simulink model "high_level"  (R2016b)
settings: Solver=FixedStepAuto  StartTime=0.0  StopTime=inf  FixedStep=0.05  RelTol=1e-3
values from neighbouring files (symbols this model uses):
  Ki = 0.2    [run.m]    (also in run_with_python.m)
  Kia = 20    [run.m]    (also in run_with_python.m = -0.3)
  kiax = 20    [run.m]    (also in run_with_python.m)
  Kix = 0.2    [run.m]    (also in run_with_python.m)
  Kp = 11.9    [run.m]    (also in run_with_python.m = 6)
  Kpa = 4    [run.m]    (also in run_with_python.m)
  Kpax = 4    [run.m]    (also in run_with_python.m)
  Kpx = 11.9    [run.m]    (also in run_with_python.m)
  START_COURSE = 1    [run.m]    (also in run_with_python.m)
  total_waypoints = length(xwaypoints)    [run.m]    (also in run_with_python.m = length(waypoints_list))
  TxBreak = 0    [run.m]    (also in run_with_python.m)
  TxCoulomb = 2.5    [run.m]    (also in run_with_python.m)
  TxVisc = 49.1750    (= 49.175)    [run.m]    (also in run_with_python.m)
  TyBreak = 0    [run.m]    (also in run_with_python.m)
  TyCoulomb = 1.8    [run.m]    (also in run_with_python.m)
  xwaypoints = targets(:,1)/100    [run.m]
  xZero = 0    [run.m]    (also in run_with_python.m)
  ywaypoints = targets(:,2)/100    [run.m]
  yZero = 0.    (= 0)    [run.m]    (also in run_with_python.m)
undefined symbols (not defined in the file or in its folder): m, MR, TzBreak, TzCoulomb, X, xRange, Y, yRange, Z, zRange, zZero
undefined symbols (not defined in the file): M, TorqueMultX, TorqueMultY, TorqueMultZ, TxTrans, TyTrans, TyVisc, TzTrans, TzVisc
libraries: sm_lib x146, fl_lib x62, nesl_utility x24, elec_lib x9, simulink x6, sm_double_wishbone_suspension_lib x4, aerolibtransform2 x1
(part 1 of 14)
settings Model: Creator=nadeen  LastModifiedBy=nadeen
settings DataIOCC: ReturnWorkspaceOutputs=on

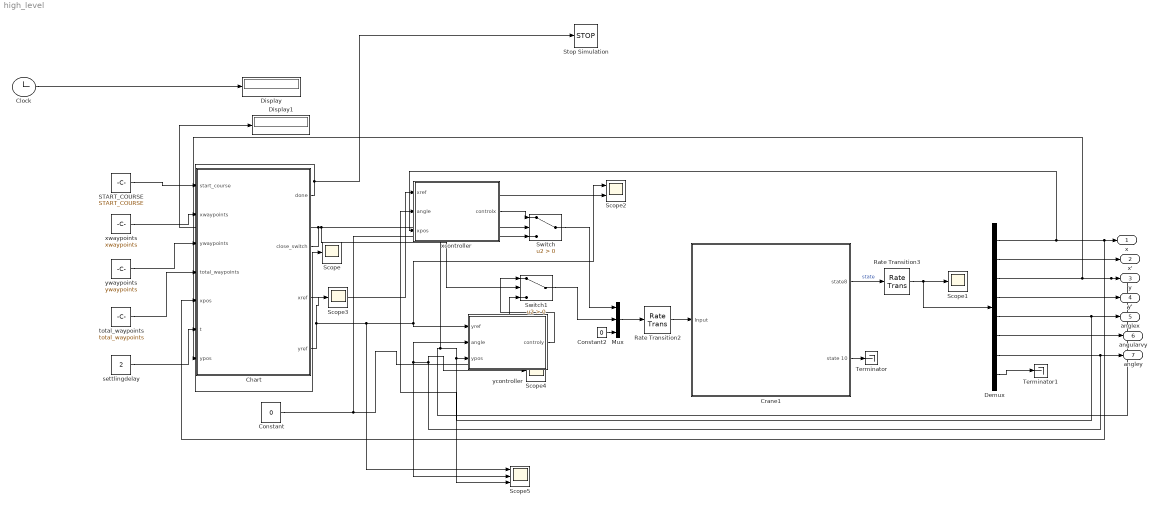
== system high_level ==
  Chart : Stateflow chart  TreatAsAtomicUnit=on
  Clock : Clock
  Constant : Constant  Value=0
  Constant2 : Constant  Value=0
  Crane1 : Subsystem  mask{penduMass=m, cartMass=M, MR=MR, xRange=xRange, yRange=yRange, zRange=zRange, xZero=xZero, yZero=yZero, zZero=zZero, TxBreak=TxBreak, TxCoulomb=TxCoulomb, TxVisc=TxVisc, TxTrans=TxTrans, TyBreak=TyBreak, TyCoulomb=TyCoulomb, TyVisc=TyVisc, TyTrans=TyTrans, TzBreak=TzBreak, TzCoulomb=TzCoulomb, TzVisc=TzVisc, TzTrans=TzTrans, Ux=TorqueMultX, Uy=TorqueMultY, Uz=TorqueMultZ}
      mask prompts: penduMass "Pendulum Mass (Kg)"; cartMass "Mass of the cart (Kg)"; MR "Mass of the rail (Kg)"; TxBreak "BreakAwayFriction"; TxCoulomb "Coulomb Friction"; TxVisc "Viscous friction"; TxTrans "Transition coeff"; TyBreak "BreakAwayFriction"; TyCoulomb "Coulomb Friction"; TyVisc "Viscous friction"; TyTrans "Transition coeff"; TzBreak "BreakAwayFriction"; TzCoulomb "Coulomb Friction"; TzVisc "Viscous friction"; TzTrans "Transition coeff"; Ux "Rail motor multiplier (X)"; Uy "Cart motor multiplier (Y)"; Uz "String motor multiplier (Z)"
      mask init:
      | %mass lowSat
      | penduMass=max(penduMass,1e-3);
      | cartMass=max(cartMass,1e-3);
      | MR=max(MR,1e-3);
      | 
      | %zeros saturated
      | xZero=max(xZero,xRange(1));
      | xZero=min(xZero,xRange(2));
      | 
      | yZero=max(yZero,yRange(1));
      | yZero=min(yZero,yRange(2));
      | 
      | zZero=max(zZero,zRange(1));
      | zZero=min(zZero,zRange(2));
      mask DialogControl DescGroupVar Prompt: 3D Crane Simscape model
      mask Display:
